simulink model "WF_offshore"  (R2024a)
settings: Solver=VariableStepAuto  StartTime=0  StopTime=1  RelTol=1e-3
values from neighbouring files (symbols this model uses):
  c_c = 0.177e-6    (= 1.77e-07)    [WF_onshore_SSO_GFL.m]    (also in WF_physical_param_offshore_supersynchronous.m = cable_220(i,6)*1e-9; WF_physical_param_onshore_SSO_020625.m = cable_220(i,6)*1e-9; initialize_params_agg.m)
  c_c_eff = c_c*n_cables    [WF_onshore_SSO_GFL.m]    (also in WF_physical_param_offshore_supersynchronous.m; WF_physical_param_onshore_SSO_020625.m; initialize_params_agg.m)
  cvtr = initialize_NR_VSC_GF(cvtr)    [NR_steadystate_VSC_GF.m]    (also in WF_onshore_SSO_GFL.m = setfield(cvtr,'parameters', p_vary.name,p_vary.val(i)); WF_physical_param_offshore_supersynchronous.m = setfield(cvtr,'parameters', p_vary.name,p_vary.val(i)); WF_physical_param_onshore_SSO_020625.m = setfield(cvtr,'parameters', p_vary.name,p_vary.val(i)); impedance_WT_blackbox.m = base_values(cvtr))
  D_C = 10:4:100    [WF_onshore_SSO_GFL.m]    (also in WF_parameter_variation.m = 10:4:150; WF_physical_param.m = 10:4:150; WF_physical_param_offshore_supersynchronous.m = 50; WF_physical_param_onshore_SSO_020625.m = 50)
  enable_pll = 1    [impedance_WT_agg.m]    (also in initialize_WT_agg.m; initialize_WT_default_gfl.m; initialize_WT_default_offshore_super.m)
  f1 = 50    [WF_onshore_SSO_GFL.m]    (also in WF_physical_param_offshore_supersynchronous.m; WF_physical_param_onshore_SSO_020625.m; initialize_params_agg.m)
  i = 1    [WF_physical_param_offshore_supersynchronous.m]    (also in WF_physical_param_onshore_SSO_020625.m)
  L = inv(R)    [participation_factors_VSC_GF.m]
  l_c = 0.386e-3    (= 0.000386)    [WF_onshore_SSO_GFL.m]    (also in WF_physical_param_offshore_supersynchronous.m = cable_220(i,5)*1e-3; WF_physical_param_onshore_SSO_020625.m = cable_220(i,5)*1e-3; initialize_params_agg.m)
  l_c_eff = l_c/n_cables    [WF_onshore_SSO_GFL.m]    (also in WF_physical_param_offshore_supersynchronous.m; WF_physical_param_onshore_SSO_020625.m; initialize_params_agg.m)
  L_comp = sqrt(2)*l_comp*(Z_b_G/(2*pi*f1))    [WF_physical_param.m]    (also in WF_physical_param_offshore_supersynchronous.m = sqrt(2)*((1/(c_c_eff/2*D_C*2*pi*f1))-(l_tf_wf*(Z_b_G)+(l_c_e; WF_physical_param_onshore_SSO_020625.m = sqrt(2)*((1/(c_c_eff/2*D_C*2*pi*f1))-(l_tf_wf*(Z_b_G)+(l_c_e; initialize_params_agg.m)
  l_OH = 0.2    [WF_onshore_SSO_GFL.m]    (also in WF_physical_param_offshore_supersynchronous.m = 0.1; WF_physical_param_onshore_SSO_020625.m = 0.1; initialize_params_agg.m = 0.1)
  l_tf_wf = tf_params(2,2)    [IM_WF_agg.m]    (also in WF_onshore_SSO_GFL.m = 0.05; WF_physical_param_offshore_supersynchronous.m = 0.05; WF_physical_param_onshore_SSO_020625.m = 0.05; initialize_params_agg.m = 0.05)
  l_tf_wt = tf_params(1,2)    [IM_WF_agg.m]    (also in WF_onshore_SSO_GFL.m = 0.0392; WF_physical_param_offshore_supersynchronous.m = 0.0392; WF_physical_param_onshore_SSO_020625.m = 0.0392; initialize_params_agg.m = 0.0392)
  Lg = p_vary(i)*((Z_b_G/(2*pi*f1)))    [WF_onshore_SSO_GFL.m]    (also in WF_physical_param_offshore_supersynchronous.m; WF_physical_param_onshore_SSO_020625.m; initialize_params_agg.m = 0.1*((Z_b_G/(2*pi*f1))))
  Lg1 = Lg    [WF_physical_param_offshore_supersynchronous.m]    (also in WF_physical_param_onshore_SSO_020625.m)
  Lg2 = Lg    [WF_physical_param_offshore_supersynchronous.m]    (also in WF_physical_param_onshore_SSO_020625.m)
  r_c = 27e-3    (= 0.027)    [WF_onshore_SSO_GFL.m]    (also in WF_physical_param_offshore_supersynchronous.m = cable_220(i,4)*1e-3; WF_physical_param_onshore_SSO_020625.m = cable_220(i,4)*1e-3; initialize_params_agg.m)
  r_c_eff = r_c/n_cables    [WF_onshore_SSO_GFL.m]    (also in WF_physical_param_offshore_supersynchronous.m; WF_physical_param_onshore_SSO_020625.m; initialize_params_agg.m)
  r_diss = .1    (= 0.1)    [WF_physical_param_offshore_supersynchronous.m]    (also in WF_physical_param_onshore_SSO_020625.m; calculate_WF.m; initialize_params_agg.m)
  r_OH = 0.02    [WF_onshore_SSO_GFL.m]    (also in WF_physical_param_offshore_supersynchronous.m = 0.01; WF_physical_param_onshore_SSO_020625.m = 0.01; initialize_params_agg.m)
  r_tf_wf = tf_params(2,1)    [IM_WF_agg.m]    (also in WF_onshore_SSO_GFL.m = 0.005; WF_physical_param_offshore_supersynchronous.m = 0.005; WF_physical_param_onshore_SSO_020625.m = 0.005; initialize_params_agg.m = 0.005)
  r_tf_wt = tf_params(1,1)    [IM_WF_agg.m]    (also in WF_onshore_SSO_GFL.m = 0.0056; WF_physical_param_offshore_supersynchronous.m = 0.0056; WF_physical_param_onshore_SSO_020625.m = 0.0056; initialize_params_agg.m = 0.0056)
  Rg = rg*Z_b_G    [WF_onshore_SSO_GFL.m]    (also in WF_physical_param_offshore_supersynchronous.m; WF_physical_param_onshore_SSO_020625.m; initialize_params_agg.m = 0.01*Z_b_G)
  Sb_WF = (3*1)*5e6    (= 15000000)    [WF_onshore_SSO_GFL.m]    (also in WF_physical_param_offshore_supersynchronous.m; WF_physical_param_onshore_SSO_020625.m; impedance_WT_blackbox.m = n_t*Sb_WT; initialize_params_agg.m = 1000000000)
  Sb_WT = 5e6    (= 5000000)    [IM_WF.m]    (also in WF_onshore_SSO_GFL.m; WF_physical_param_offshore_supersynchronous.m; WF_physical_param_onshore_SSO_020625.m; initialize_params_agg.m)
  selector_current_reference = 3    [impedance_WT_agg.m]    (also in initialize_WT_agg.m; initialize_WT_default_gfl.m; initialize_WT_default_offshore_super.m)
  selector_omega_reference = 1    [impedance_WT_agg.m]    (also in initialize_WT_agg.m; initialize_WT_default_gfl.m; initialize_WT_default_offshore_super.m)
  V_coll = 33e3    (= 33000)    [WF_onshore_SSO_GFL.m]    (also in WF_physical_param_offshore_supersynchronous.m; WF_physical_param_onshore_SSO_020625.m; initialize_params_agg.m)
  V_trans = 220e3    (= 220000)    [WF_onshore_SSO_GFL.m]    (also in WF_physical_param_offshore_supersynchronous.m; WF_physical_param_onshore_SSO_020625.m; initialize_params_agg.m)
  Z_b_G = (V_trans/sqrt(3/2))^2/Sb_WF    [WF_onshore_SSO_GFL.m]    (also in WF_physical_param_offshore_supersynchronous.m = (V_b_trans)^2/Sb_WF; WF_physical_param_onshore_SSO_020625.m = (V_b_trans)^2/Sb_WF; initialize_params_agg.m = (V_b_trans)^2/Sb_WF)
undefined symbols (not defined in the file or in its folder): opts, R
libraries: spsSeriesRLCBranchLib x105, simulink_extras x104, simulink x52, spsThreePhaseVIMeasurementLib x42, spsControlledVoltageSourceLib x42, spsGroundLib x41, spsThreePhaseTransformerTwoWindingsLib x14, powerlib_extras x13, spsVariableInductorLib x9, spsIdealSwitchLib x6, spsVariableCapacitorLib x6, spsThreePhaseSeriesRLCBranchLib x4
(part 1 of 13)
settings Model: Creator=andrsmit  LastModifiedBy=andrsmit
settings DataIOCC: InitialState=op.xFinal  SaveFinalState=on  SaveOperatingPoint=on

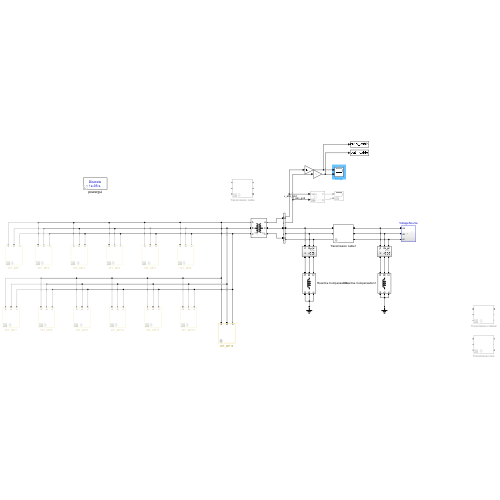
[thumbnail: Simulink's stored preview of the top-level diagram]
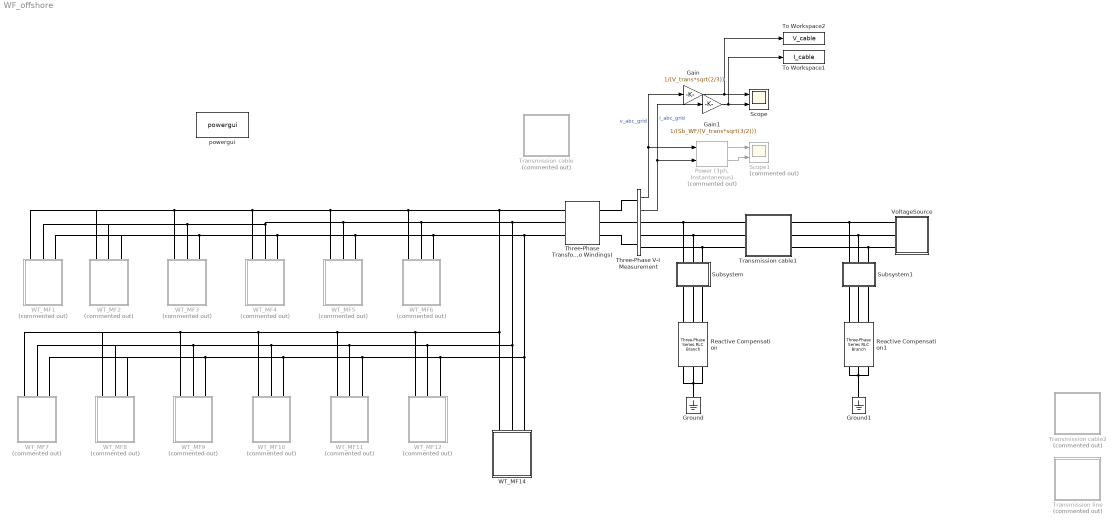
== system WF_offshore ==
  Gain : Gain  Gain=1/(V_trans*sqrt(2/3))
  Gain1 : Gain  Gain=1/(Sb_WF/(V_trans*sqrt(3/2)))
  Ground : spsGroundLib/Ground  LConnTagsString=a
  Ground1 : spsGroundLib/Ground  LConnTagsString=a
  "Power (3ph, Instantaneous)" : spsPower3phInstantaneousLib/Power (3ph, Instantaneous)  Commented=on
  Reactive Compensation : spsThreePhaseSeriesRLCBranchLib/Three-Phase Series RLC Branch  LConnTagsString=A|B|C  RConnTagsString=A|B|C  BranchType=L  Resistance=100  Inductance=L_comp  Capacitance=1e-6  Measurements=None
  Reactive Compensation1 : spsThreePhaseSeriesRLCBranchLib/Three-Phase Series RLC Branch  LConnTagsString=A|B|C  RConnTagsString=A|B|C  BranchType=L  Resistance=100  Inductance=L_comp  Capacitance=1e-6  Measurements=None
  Scope : Scope  NumInputPorts=2
  Scope1 : Scope  Commented=on  NumInputPorts=2
  Subsystem : Subsystem
  Subsystem1 : Subsystem
  Three-Phase Transformer (Two Windings) : spsThreePhaseTransformerTwoWindingsLib/Three-Phase Transformer (Two Windings)  Winding1Connection=Yg  Winding2Connection=Yg  CoreType=Three single-phase transformers  SetSaturation=off  Hysteresis=off  DataFile='hysteresis'  SetInitialFlux=off  Measurements=None  UNITS=pu  NominalPower=[Sb_WF , 50 ]  Winding1=[V_coll , r_tf_wf/2, l_tf_wf/2]  Winding2=[V_trans, r_tf_wf/2, l_tf_wf/2]  Rm=5000  Lm=0  L0=0.5  Saturation=[ 0,0 ; 0.0024,1.2 ; 1.0,1.52 ]  InitialFluxes=[ 0.8 , -0.8 , 0.7 ]  BreakLoop=off  DiscreteSolver=Trapezoidal iterative  DataType=off  TransfoNumber=1
  Three-Phase V-I Measurement : spsThreePhaseVIMeasurementLib/Three-Phase V-I Measurement  VoltageMeasurement=phase-to-ground  SetLabelV=off  LabelV=Vabc  Vpu=off  VpuLL=off  CurrentMeasurement=yes  SetLabelI=off  LabelI=Iabc  Ipu=off  Pbase=100e6  Vbase=500e3  OutputType=Complex  PhasorSimulation=off  PSBequivalent=0
  To Workspace1 : ToWorkspace  VariableName=I_cable  SaveFormat=Structure With Time  SampleTime=-1
      settings: MaxDataPoints=1e5
  To Workspace2 : ToWorkspace  VariableName=V_cable  SaveFormat=Structure With Time  SampleTime=-1
      settings: MaxDataPoints=1e6
  Transmission cable : Subsystem  Commented=on  mask{D=D_C, r=r_c, l=l_c, c=c_c}
      mask prompts: D "Distance (km)"; r "Resistance/km (Ohms/km)"; l "Inductance/km (H/km)"; c "Capacitance/km (F/km)"
      mask DialogControl DescTextVar Prompt: Single PI-line cable model, with no coupling/connection between phases
  Transmission cable1 : Subsystem  mask{D=D_C, r=r_c_eff, l=l_c_eff, c=c_c_eff}
      mask prompts: D "Distance (km)"; r "Resistance/km (Ohms/km)"; l "Inductance/km (H/km)"; c "Capacitance/km (F/km)"
      mask DialogControl DescTextVar Prompt: Single PI-line cable model, with no coupling/connection between phases
  Transmission cable2 : Subsystem  Commented=on  mask{D=D_C, r=r_c_eff, l=l_c_eff, c=c_c_eff}
      mask prompts: D "Distance (km)"; r "Resistance/km (Ohms/km)"; l "Inductance/km (H/km)"; c "Capacitance/km (F/km)"
      mask DialogControl DescTextVar Prompt: Single PI-line cable model, with no coupling/connection between phases
  Transmission line : Subsystem  Commented=on  mask{r=r_OH*Z_b_G, l=l_OH*(Z_b_G/(2*pi*f1))}
      mask prompts: r "Resistance (Ohms)"; l "Inductance (H)"
      mask DialogControl DescTextVar Prompt: Single PI-line cable model, with no coupling/connection between phases
  VoltageSource : Subsystem
  WT_MF1 : Subsystem  Commented=on  mask{cvtr=cvtr}
      mask prompts: cvtr "converter name"
  WT_MF10 : Subsystem  Commented=on  mask{cvtr=cvtr}
      mask prompts: cvtr "converter name"
  WT_MF11 : Subsystem  Commented=on  mask{cvtr=cvtr}
      mask prompts: cvtr "converter name"
  WT_MF12 : Subsystem  Commented=on  mask{cvtr=cvtr}
      mask prompts: cvtr "converter name"
  WT_MF14 : Subsystem  mask{cvtr=cvtr}
      mask prompts: cvtr "converter name"
  WT_MF2 : Subsystem  Commented=on  mask{cvtr=cvtr}
      mask prompts: cvtr "converter name"
  WT_MF3 : Subsystem  Commented=on  mask{cvtr=cvtr}
      mask prompts: cvtr "converter name"
  WT_MF4 : Subsystem  Commented=on  mask{cvtr=cvtr}
      mask prompts: cvtr "converter name"
  WT_MF5 : Subsystem  Commented=on  mask{cvtr=cvtr}
      mask prompts: cvtr "converter name"
  WT_MF6 : Subsystem  Commented=on  mask{cvtr=cvtr}
      mask prompts: cvtr "converter name"
  WT_MF7 : Subsystem  Commented=on  mask{cvtr=cvtr}
      mask prompts: cvtr "converter name"
  WT_MF8 : Subsystem  Commented=on  mask{cvtr=cvtr}
      mask prompts: cvtr "converter name"
  WT_MF9 : Subsystem  Commented=on  mask{cvtr=cvtr}
      mask prompts: cvtr "converter name"
  powergui : spspowerguiLib/powergui  Priority=2  SimulationMode=Discrete  SampleTime=cvtr.parameters.Ts  frequency=60  Iterations=50  frequencyindice=0  Pbase=100e6  ErrMax=0.0001  UnitsV=kV  UnitsW=MW  buscounter=0  FunctionMessages=off  echomessages=off  EnableUseOfTLC=off  CurrentSourceSwitches=off  DisableSnubberDevices=off  DisableRonSwitches=off  DisableVfSwitches=off  DisplayEquations=off  AutomaticDiscreteSolvers=off  SolverType=Tustin  Interpol=off  ExternalGateDelay=off  methode=off  Ts=0  x0status=blocks  SPID=off  SwTol=0  HookPort=off  NonlinearTolerance=1e-4  nMaxIteration=100  ContinueOnMaxIteration=off  RestoreLinks=warning  ResistiveCurrentMeasurement=off  Frange=logspace(0,3,50)  Ylog=off  Xlog=off  ShowGrid=off  save=off  variable=ZData  structure=0  ZoomFFT=on  StartTime=0.0  cycles=1  DisplayStyle=1  fundamental=60  FreqAxis=off  MaxFrequency=1000  frequencyindicesteady=1  RmsSteady=1  display=off
  wires:
  Three-Phase V-I Measurement/1 -> Gain/1, "Power (3ph, Instantaneous)"/1  "v_abc_grid"
  Three-Phase V-I Measurement/2 -> "Power (3ph, Instantaneous)"/2, Gain1/1  "i_abc_grid"
  Gain/1 -> To Workspace2/1, Scope/1
  Gain1/1 -> To Workspace1/1, Scope/2
  "Power (3ph, Instantaneous)"/1 -> Scope1/1
  "Power (3ph, Instantaneous)"/2 -> Scope1/2
  connections:
  Three-Phase Transformer (Two Windings)/RConn1 -- Three-Phase V-I Measurement/LConn1
  Three-Phase Transformer (Two Windings)/RConn2 -- Three-Phase V-I Measurement/LConn2
  Three-Phase Transformer (Two Windings)/RConn3 -- Three-Phase V-I Measurement/LConn3
  WT_MF4/RConn1 -- WT_MF3/RConn1 -- WT_MF2/RConn1 -- WT_MF1/RConn1 -- WT_MF5/RConn1 -- WT_MF6/RConn1 -- WT_MF12/RConn1 -- WT_MF11/RConn1 -- WT_MF10/RConn1 -- WT_MF9/RConn1 -- WT_MF7/RConn1 -- WT_MF8/RConn1 -- WT_MF14/RConn1 -- Three-Phase Transformer (Two Windings)/LConn1
  WT_MF4/RConn2 -- WT_MF3/RConn2 -- WT_MF2/RConn2 -- WT_MF1/RConn2 -- WT_MF5/RConn2 -- WT_MF6/RConn2 -- Three-Phase Transformer (Two Windings)/LConn2 -- WT_MF14/RConn2 -- WT_MF12/RConn2 -- WT_MF11/RConn2 -- WT_MF10/RConn2 -- WT_MF9/RConn2 -- WT_MF7/RConn2 -- WT_MF8/RConn2
  Three-Phase Transformer (Two Windings)/LConn3 -- WT_MF14/RConn3 -- WT_MF12/RConn3 -- WT_MF11/RConn3 -- WT_MF10/RConn3 -- WT_MF9/RConn3 -- WT_MF7/RConn3 -- WT_MF8/RConn3 -- WT_MF6/RConn3 -- WT_MF5/RConn3 -- WT_MF4/RConn3 -- WT_MF3/RConn3 -- WT_MF2/RConn3 -- WT_MF1/RConn3
  Transmission cable1/RConn1 -- Subsystem1/LConn1 -- VoltageSource/RConn1
  VoltageSource/RConn2 -- Subsystem1/LConn2 -- Transmission cable1/RConn2
  Transmission cable1/LConn3 -- Subsystem/LConn3 -- Three-Phase V-I Measurement/RConn3
  Ground/LConn1 -- Reactive Compensation/RConn1 -- Reactive Compensation/RConn3 -- Reactive Compensation/RConn2
  Reactive Compensation1/RConn3 -- Reactive Compensation1/RConn1 -- Ground1/LConn1 -- Reactive Compensation1/RConn2
  Transmission cable1/RConn3 -- Subsystem1/LConn3 -- VoltageSource/RConn3
  Subsystem/RConn2 -- Reactive Compensation/LConn2
  Subsystem/RConn1 -- Reactive Compensation/LConn1
  Transmission cable1/LConn2 -- Subsystem/LConn2 -- Three-Phase V-I Measurement/RConn2
  Subsystem/RConn3 -- Reactive Compensation/LConn3
  Transmission cable1/LConn1 -- Three-Phase V-I Measurement/RConn1 -- Subsystem/LConn1
  Subsystem1/RConn3 -- Reactive Compensation1/LConn3
  Subsystem1/RConn1 -- Reactive Compensation1/LConn1
  Subsystem1/RConn2 -- Reactive Compensation1/LConn2

== system WF_offshore/Subsystem ==
  Ideal Switch : spsIdealSwitchLib/Ideal Switch  Ron=R_comp  Lon=0  IC=0  Rs=r_diss*Z_b_G  Cs=inf  Measurements=off
  Ideal Switch1 : spsIdealSwitchLib/Ideal Switch  Ron=R_comp  Lon=0  IC=0  Rs=r_diss*Z_b_G  Cs=inf  Measurements=off
  Ideal Switch2 : spsIdealSwitchLib/Ideal Switch  Ron=R_comp  Lon=0  IC=0  Rs=r_diss*Z_b_G  Cs=inf  Measurements=off
  Step : Step  Time=0.5  SampleTime=0
  Three-Phase Series RLC Branch : spsThreePhaseSeriesRLCBranchLib/Three-Phase Series RLC Branch  Commented=on  LConnTagsString=A|B|C  RConnTagsString=A|B|C  BranchType=RLC  Resistance=1  Inductance=1e-3  Capacitance=1e-6  Measurements=None
  " A" : PMIOPort  Side=Left
  " B" : PMIOPort  Port=2  Side=Left
  " C" : PMIOPort  Port=3  Side=Left
  "  a" : PMIOPort  Port=4  Side=Right
  "  b" : PMIOPort  Port=5  Side=Right
  "  c" : PMIOPort  Port=6  Side=Right
  wires:
  Step/1 -> Ideal Switch2/1, Ideal Switch1/1, Ideal Switch/1
  connections:
  "  a"/RConn1 -- Ideal Switch/RConn1
  Ideal Switch2/LConn1 -- " C"/RConn1
  Ideal Switch2/RConn1 -- "  c"/RConn1
  " A"/RConn1 -- Ideal Switch/LConn1
  Ideal Switch1/RConn1 -- "  b"/RConn1
  Ideal Switch1/LConn1 -- " B"/RConn1

== system WF_offshore/Subsystem1 ==
  Ideal Switch : spsIdealSwitchLib/Ideal Switch  Ron=R_comp  Lon=0  IC=0  Rs=r_diss*Z_b_G  Cs=inf  Measurements=off
  Ideal Switch1 : spsIdealSwitchLib/Ideal Switch  Ron=R_comp  Lon=0  IC=0  Rs=r_diss*Z_b_G  Cs=inf  Measurements=off
  Ideal Switch2 : spsIdealSwitchLib/Ideal Switch  Ron=R_comp  Lon=0  IC=0  Rs=r_diss*Z_b_G  Cs=inf  Measurements=off
  Step : Step  Time=0.5  Before=1  SampleTime=0
  Three-Phase Series RLC Branch : spsThreePhaseSeriesRLCBranchLib/Three-Phase Series RLC Branch  Commented=on  LConnTagsString=A|B|C  RConnTagsString=A|B|C  BranchType=RLC  Resistance=1  Inductance=1e-3  Capacitance=1e-6  Measurements=None
  " A" : PMIOPort  Side=Left
  " B" : PMIOPort  Port=2  Side=Left
  " C" : PMIOPort  Port=3  Side=Left
  "  a" : PMIOPort  Port=4  Side=Right
  "  b" : PMIOPort  Port=5  Side=Right
  "  c" : PMIOPort  Port=6  Side=Right
  wires:
  Step/1 -> Ideal Switch/1, Ideal Switch1/1, Ideal Switch2/1
  connections:
  Ideal Switch1/LConn1 -- " B"/RConn1
  Ideal Switch1/RConn1 -- "  b"/RConn1
  " A"/RConn1 -- Ideal Switch/LConn1
  Ideal Switch2/RConn1 -- "  c"/RConn1
  Ideal Switch2/LConn1 -- " C"/RConn1
  "  a"/RConn1 -- Ideal Switch/RConn1

== system WF_offshore/Transmission cable ==
  Pi Section Line : spsPiSectionLineLib/Pi Section Line  LConnTagsString=1  RConnTagsString=1  Phases=1  PiSections=1  Length=D  Frequency=50  Resistance=r  Inductance=l  Capacitance=c  SpecifyConductance=off  Conductance=0  Measurements=None  Measurements2=None
      settings: LibrarySourceBlock=sps_lib/Power Grid Elements/Pi Section Line
  Pi Section Line1 : spsPiSectionLineLib/Pi Section Line  LConnTagsString=1  RConnTagsString=1  Phases=1  PiSections=1  Length=D  Frequency=50  Resistance=r  Inductance=l  Capacitance=c  SpecifyConductance=off  Conductance=0  Measurements=None  Measurements2=None
      settings: LibrarySourceBlock=sps_lib/Power Grid Elements/Pi Section Line
  Pi Section Line2 : spsPiSectionLineLib/Pi Section Line  LConnTagsString=1  RConnTagsString=1  Phases=1  PiSections=1  Length=D  Frequency=50  Resistance=r  Inductance=l  Capacitance=c  SpecifyConductance=off  Conductance=0  Measurements=None  Measurements2=None
      settings: LibrarySourceBlock=sps_lib/Power Grid Elements/Pi Section Line
  A : PMIOPort  Side=Left
  a : PMIOPort  Port=2  Side=Right
  B : PMIOPort  Port=3  Side=Left
  b : PMIOPort  Port=4  Side=Right
  C : PMIOPort  Port=5  Side=Left
  c : PMIOPort  Port=6  Side=Right
  connections:
  Pi Section Line2/LConn1 -- C/RConn1
  Pi Section Line1/RConn1 -- b/RConn1
  Pi Section Line2/RConn1 -- c/RConn1
  Pi Section Line1/LConn1 -- B/RConn1
  Pi Section Line/LConn1 -- A/RConn1
  a/RConn1 -- Pi Section Line/RConn1

== system WF_offshore/Transmission cable1 ==
  Subsystem : Subsystem
  Subsystem1 : Subsystem
  Subsystem2 : Subsystem
  A : PMIOPort  Side=Left
  a : PMIOPort  Port=2  Side=Right
  B : PMIOPort  Port=3  Side=Left
  b : PMIOPort  Port=4  Side=Right
  C : PMIOPort  Port=5  Side=Left
  c : PMIOPort  Port=6  Side=Right
  connections:
  Subsystem/RConn1 -- a/RConn1
  Subsystem/LConn1 -- A/RConn1
  Subsystem1/LConn1 -- B/RConn1
  Subsystem2/RConn1 -- c/RConn1
  Subsystem1/RConn1 -- b/RConn1
  Subsystem2/LConn1 -- C/RConn1

== system WF_offshore/Transmission cable2 ==
  Subsystem : Subsystem
  Subsystem1 : Subsystem
  Subsystem2 : Subsystem
  A : PMIOPort  Side=Left
  a : PMIOPort  Port=2  Side=Right
  B : PMIOPort  Port=3  Side=Left
  b : PMIOPort  Port=4  Side=Right
  C : PMIOPort  Port=5  Side=Left
  c : PMIOPort  Port=6  Side=Right
  connections:
  Subsystem2/LConn1 -- C/RConn1
  Subsystem1/RConn1 -- b/RConn1
  Subsystem2/RConn1 -- c/RConn1
  Subsystem1/LConn1 -- B/RConn1
  Subsystem/LConn1 -- A/RConn1
  Subsystem/RConn1 -- a/RConn1

== system WF_offshore/Transmission line ==
  Series RLC Branch1 : spsSeriesRLCBranchLib/Series RLC Branch  LConnTagsString=__new0  RConnTagsString=__new0  BranchType=RL  Resistance=r  Inductance=l  SetiL0=off  InitialCurrent=0  Capacitance=1e-6  Setx0=off  InitialVoltage=0  Measurements=None
  Series RLC Branch3 : spsSeriesRLCBranchLib/Series RLC Branch  LConnTagsString=__new0  RConnTagsString=__new0  BranchType=RL  Resistance=r  Inductance=l  SetiL0=off  InitialCurrent=0  Capacitance=1e-6  Setx0=off  InitialVoltage=0  Measurements=None
  Series RLC Branch4 : spsSeriesRLCBranchLib/Series RLC Branch  LConnTagsString=__new0  RConnTagsString=__new0  BranchType=RL  Resistance=r  Inductance=l  SetiL0=off  InitialCurrent=0  Capacitance=1e-6  Setx0=off  InitialVoltage=0  Measurements=None
  A : PMIOPort  Side=Left
  a : PMIOPort  Port=2  Side=Right
  B : PMIOPort  Port=3  Side=Left
  b : PMIOPort  Port=4  Side=Right
  C : PMIOPort  Port=5  Side=Left
  c : PMIOPort  Port=6  Side=Right
  connections:
  Series RLC Branch1/LConn1 -- a/RConn1
  B/RConn1 -- Series RLC Branch3/RConn1
  Series RLC Branch4/LConn1 -- c/RConn1
  Series RLC Branch3/LConn1 -- b/RConn1
  C/RConn1 -- Series RLC Branch4/RConn1
  A/RConn1 -- Series RLC Branch1/RConn1

== system WF_offshore/VoltageSource ==
  1 : spsThreePhaseVIMeasurementLib/Three-Phase V-I Measurement  VoltageMeasurement=phase-to-ground  SetLabelV=off  LabelV=Vabc_1  Vpu=off  VpuLL=off  CurrentMeasurement=yes  SetLabelI=off  LabelI=Iabc_1  Ipu=off  Pbase=100e6  Vbase=Bus(1,2)*1e3  OutputType=Complex  PhasorSimulation=off  PSBequivalent=0
  40 : spsThreePhaseVIMeasurementLib/Three-Phase V-I Measurement  VoltageMeasurement=phase-to-ground  SetLabelV=off  LabelV=Vabc_1  Vpu=off  VpuLL=off  CurrentMeasurement=yes  SetLabelI=off  LabelI=Iabc_1  Ipu=off  Pbase=100e6  Vbase=Bus(1,2)*1e3  OutputType=Complex  PhasorSimulation=off  PSBequivalent=0
  Add2 : Sum
  Add4 : Sum
  Add5 : Sum
  Gain : Gain  Commented=on  Gain=1/(V_trans*sqrt(2/3))
  Gain1 : Gain  Gain=cvtr.pu.Omegab
  Gain2 : Gain  Commented=on  Gain=1/(Sb_WF/(V_trans*sqrt(3/2)))
  Gain3 : Gain  Commented=on  Gain=1/(V_trans*sqrt(2/3))
  Gain4 : Gain  Commented=on  Gain=1/(Sb_WF/(V_trans*sqrt(3/2)))
  Integrator2 : Integrator  InitialConditionSource=external
  Inverse Park1 : Subsystem
  "Power (3ph, Instantaneous)" : spsPower3phInstantaneousLib/Power (3ph, Instantaneous)
  "Power (3ph, Instantaneous)1" : spsPower3phInstantaneousLib/Power (3ph, Instantaneous)  Commented=on
  Product2 : Product
  Product3 : Product
  Scope : Scope  Commented=on  NumInputPorts=2
  Scope1 : Scope  NumInputPorts=2
  Scope2 : Scope  Commented=on  NumInputPorts=2
  Scope3 : Scope  Commented=on  NumInputPorts=2
  Sine Wave1 : Sin  Commented=on  Amplitude=0.01  Frequency=20*2*pi  SampleTime=0
  Step1 : Step  Commented=on  Time=0.1  After=1e-4  SampleTime=0
  Subsystem1 : Subsystem
  Subsystem2 : Subsystem
  Sum2 : Sum  Inputs=++|
  Sum3 : Sum  Inputs=|++
  To Workspace5 : ToWorkspace  Commented=on  VariableName=V_g  SaveFormat=Structure With Time  SampleTime=-1
      settings: MaxDataPoints=2000000
  To Workspace6 : ToWorkspace  Commented=on  VariableName=I_g  SaveFormat=Structure With Time  SampleTime=-1
      settings: MaxDataPoints=2000000
  d_input1 : Constant  Value=0  SampleTime=opts.inp.ts
  delta1 : Constant  Value=0
  dvnd1 : Constant  Value=0  SampleTime=opts.inp.ts
  dvnq1 : Constant  Value=0  SampleTime=opts.inp.ts
  grid inductance : Subsystem  Commented=on
  grid inductance+line : Subsystem  Commented=on
  grid inductance1 : Subsystem  Commented=on
  grid inductance2 : Subsystem
  io5 : Constant  Value=cvtr.ss.vnd0
  io6 : Constant  Value=V_trans*sqrt(2/3)
  io7 : Constant  Value=cvtr.ss.vnq0
  io8 : Constant  Value=1i
  io9 : Constant  Commented=on  Value=cvtr.pu.Vb*(cvtr.ss.vnd0+i*cvtr.ss.vnq0)
  w1 : Constant  Value=cvtr.parameters.Omegag*cvtr.pu.Omegab
  va : PMIOPort  Side=Right
  vb : PMIOPort  Port=2  Side=Right
  vc : PMIOPort  Port=3  Side=Right
  tag scope: d_input=global, dvnd=global, dvnq=global
  wires:
  40/2 -> Gain2/1, To Workspace6/1, "Power (3ph, Instantaneous)"/2
  40/1 -> Gain/1, To Workspace5/1, "Power (3ph, Instantaneous)"/1
  Integrator2/1 -> Inverse Park1/2(delta)
  io5/1 -> Add5/2  "vnd0"
  Add4/1 -> Product3/1  "vnq"
  Subsystem2/1(x_dq) -> Inverse Park1/1(x_dq)
  Add2/1 -> Integrator2/1
  Inverse Park1/1(x_abc) -> Subsystem1/1(v_abc)
  Step1/1 -> Sum3/1
  Sum2/1 -> Product2/1
  io7/1 -> Add4/2  "vnq0"
  w1/1 -> Add2/1
  Sum3/1 -> [d_input], Gain1/1
  dvnq1/1 -> [dvnq], Add4/1  "dvnq"
  Add5/1 -> Sum2/1  "vnd"
  delta1/1 -> Integrator2/2
  dvnd1/1 -> Add5/1, [dvnd]  "dvnd"
  d_input1/1 -> Sum3/2  "d_inp"
  Product2/1 -> Subsystem2/1(x_d+ix_q)
  io8/1 -> Product3/2
  io6/1 -> Product2/2
  Product3/1 -> Sum2/2
  Gain1/1 -> Add2/2
  Gain/1 -> Scope/1
  Gain2/1 -> Scope/2
  "Power (3ph, Instantaneous)"/1 -> Scope1/1
  "Power (3ph, Instantaneous)"/2 -> Scope1/2
  "Power (3ph, Instantaneous)1"/1 -> Scope2/1
  "Power (3ph, Instantaneous)1"/2 -> Scope2/2
  1/1 -> Gain3/1, "Power (3ph, Instantaneous)1"/1
  1/2 -> Gain4/1, "Power (3ph, Instantaneous)1"/2
  Gain3/1 -> Scope3/1
  Gain4/1 -> Scope3/2
  connections:
  40/LConn1 -- vc/RConn1
  40/LConn2 -- vb/RConn1
  40/LConn3 -- va/RConn1
  grid inductance2/LConn1 -- 40/RConn3
  grid inductance2/LConn2 -- 40/RConn2
  grid inductance2/LConn3 -- 40/RConn1
  grid inductance2/RConn1 -- 1/LConn3
  grid inductance2/RConn2 -- 1/LConn2
  grid inductance2/RConn3 -- 1/LConn1
  1/RConn3 -- Subsystem1/RConn1
  1/RConn2 -- Subsystem1/RConn2
  1/RConn1 -- Subsystem1/RConn3

== system WF_offshore/WT_MF1 ==
  Control System : Subsystem  mask{Ts_control=cvtr.parameters.T_cont}
      mask prompts: Ts_control "Sample Time"
  Gain1 : Gain  Gain=1/cvtr.pu.Vb
  Gain2 : Gain  Gain=1/cvtr.pu.Ib
  Gain5 : Gain  Gain=cvtr.pu.Vb
  I_conv : ToWorkspace  VariableName=I_conv  SaveFormat=Structure With Time  SampleTime=-1
      settings: MaxDataPoints=1000000
  Inverse Park1 : Subsystem
  Scope2 : Scope  NumInputPorts=2
  Subsystem1 : Subsystem
  Subsystem6 : Subsystem
  Three-Phase Transformer (Two Windings) : spsThreePhaseTransformerTwoWindingsLib/Three-Phase Transformer (Two Windings)  Winding1Connection=Yg  Winding2Connection=Yg  CoreType=Three single-phase transformers  SetSaturation=off  Hysteresis=off  DataFile='hysteresis'  SetInitialFlux=off  Measurements=None  UNITS=pu  NominalPower=[ Sb_WT , f1]  Winding1=[cvtr.parameters.Vnr ,r_tf_wt/2 , l_tf_wt/2]  Winding2=[ V_coll , r_tf_wt/2, l_tf_wt/2]  Rm=5000  Lm=0  L0=0.5  Saturation=[ 0,0 ; 0.0024,1.2 ; 1.0,1.52 ]  InitialFluxes=[ 0.8 , -0.8 , 0.7 ]  BreakLoop=off  DiscreteSolver=Trapezoidal iterative  DataType=off  TransfoNumber=1
  Three-Phase V-I Measurement : spsThreePhaseVIMeasurementLib/Three-Phase V-I Measurement  VoltageMeasurement=phase-to-ground  SetLabelV=off  LabelV=Vabc  Vpu=off  VpuLL=off  CurrentMeasurement=yes  SetLabelI=off  LabelI=Iabc  Ipu=off  Pbase=100e6  Vbase=500e3  OutputType=Complex  PhasorSimulation=off  PSBequivalent=0
  Transformations (pu and dq) : Subsystem
  V_conv : ToWorkspace  VariableName=V_conv  SaveFormat=Structure With Time  SampleTime=-1
      settings: MaxDataPoints=1000000
  filter capacitance1 : Subsystem
      settings: PortSchema="{\"entries\":[{\"content\":{\"sides\":[{\"content\":{\"connectorIds\":[\"LConn1\",\"LConn2\",\"LConn3\"]},\"type\":\"ConnectorPlacement.EquallySpacedRectSide\",\"uuid\":\"e81be3d5-6303-4565-8ca3-afc618f21d70\"},{\"content\":{\"connectorIds\":[],\"side\":\"RIGHT\"},\"type\":\"ConnectorPlacement.EquallySpacedRectSide\",\"uuid\":\"458d9030-e614-487d-87de-3e53be7c7da4\"},{\"content\":{\"connectorIds\":[],\"side\":\"TOP\"},\"type\":\"ConnectorPlacement.EquallySpacedRectSide\",\"uuid\":\"a29d66a0-f095-498d-bb9b-96c7f47699d3\"},{\"content\":{\"connectorIds\":[\"Out1\"],\"side\":\"BOTTOM\"},\"type\":\"ConnectorPlacement.EquallySpacedRectSide\",\"uuid\":\"afc68874-c098-43f5-9b37-53a3b484513b\"}]},\"type\":\"ConnectorPlacement.EquallySpacedConnector\",\"uuid\":\"37f495dd-1c12-4bb8-af72-7ef46bbd951c\"}],\"packageUris\":[\"http://schema.mathworks.com/mf0/Connector/R2020b\"],\"version\":\"1.0\"}"
  filter inductance1 : Subsystem
      settings: PortSchema="{\"entries\":[{\"content\":{\"sides\":[{\"content\":{\"connectorIds\":[\"LConn1\",\"LConn2\",\"LConn3\"]},\"type\":\"ConnectorPlacement.EquallySpacedRectSide\",\"uuid\":\"d3d60048-9578-4fa3-8d11-9c8a66a4b1f9\"},{\"content\":{\"connectorIds\":[\"RConn1\",\"RConn2\",\"RConn3\"],\"side\":\"RIGHT\"},\"type\":\"ConnectorPlacement.EquallySpacedRectSide\",\"uuid\":\"184a2c1d-36ab-46d1-99e4-db01aa31ec94\"},{\"content\":{\"connectorIds\":[\"Out1\"],\"side\":\"TOP\"},\"type\":\"ConnectorPlacement.EquallySpacedRectSide\",\"uuid\":\"db651021-9d7f-4124-8d21-ede853163467\"}]},\"type\":\"ConnectorPlacement.EquallySpacedConnector\",\"uuid\":\"723d0964-19fd-4dbe-91e3-e4ea0bb1cca9\"}],\"packageUris\":[\"http://schema.mathworks.com/mf0/Connector/R2020b\"],\"version\":\"1.0\"}"
  a : PMIOPort  Side=Right
  b : PMIOPort  Port=2  Side=Right
  c : PMIOPort  Port=3  Side=Right
  wires:
  Control System/2(thetavsm) -> [Thetavsm]
  Control System/3(vir) -> [vir]
  Control System/1(thetapll) -> [Thetapll]
  Transformations (pu and dq)/2(il) -> Control System/2(il)  "il"
  Transformations (pu and dq)/1(io) -> Control System/1(io)  "io"
  Transformations (pu and dq)/3(p) -> Control System/3(p)  "p"
  Transformations (pu and dq)/4(q) -> Control System/4(q)  "q"
  Transformations (pu and dq)/5(vo_pll) -> Control System/5(vo_pll)  "vo_pll"
  Transformations (pu and dq)/6(vo) -> Control System/6(vo)  "vo"
  [Thetavsm] -> Transformations (pu and dq)/5(Thetavsm)
  [Thetapll] -> Transformations (pu and dq)/6(Thetapll)
  [vir] -> Gain5/1
  Subsystem6/1(x_dq) -> Inverse Park1/1(x_dq)
  Gain5/1 -> Subsystem6/1(x_d+ix_q)
  Three-Phase V-I Measurement/2 -> Gain2/1, [i_abc_grid]  "i_abc_grid"
  Inverse Park1/1(x_abc) -> Subsystem1/1(v_abc)
  Three-Phase V-I Measurement/1 -> Gain1/1, [v_abc_grid]  "v_abc_grid"
  [Thetavsm] -> Inverse Park1/2(delta)
  filter capacitance1/1(v_abc) -> [v_abc_filt]  "v_abc_filt"
  filter inductance1/1(i_abc) -> [i_abc_filt]  "i_abc_filt"
  [v_abc_grid] -> Transformations (pu and dq)/3(v_abc_grid)
  [v_abc_filt] -> Transformations (pu and dq)/4(v_abc_filt)
  [i_abc_filt] -> Transformations (pu and dq)/2(i_abc_filt)
  [i_abc_grid] -> Transformations (pu and dq)/1(i_abc_grid)
  Gain1/1 -> Scope2/1, V_conv/1
  Gain2/1 -> Scope2/2, I_conv/1
  connections:
  filter inductance1/RConn3 -- filter capacitance1/LConn3 -- Three-Phase V-I Measurement/LConn3
  filter inductance1/RConn1 -- filter capacitance1/LConn1 -- Three-Phase V-I Measurement/LConn1
  filter inductance1/RConn2 -- filter capacitance1/LConn2 -- Three-Phase V-I Measurement/LConn2
  Subsystem1/RConn1 -- filter inductance1/LConn1
  Subsystem1/RConn2 -- filter inductance1/LConn2
  Subsystem1/RConn3 -- filter inductance1/LConn3
  Three-Phase Transformer (Two Windings)/RConn1 -- a/RConn1
  Three-Phase Transformer (Two Windings)/RConn2 -- b/RConn1
  Three-Phase Transformer (Two Windings)/RConn3 -- c/RConn1
  Three-Phase Transformer (Two Windings)/LConn1 -- Three-Phase V-I Measurement/RConn1
  Three-Phase Transformer (Two Windings)/LConn2 -- Three-Phase V-I Measurement/RConn2
  Three-Phase Transformer (Two Windings)/LConn3 -- Three-Phase V-I Measurement/RConn3

== system WF_offshore/WT_MF10 ==
  Control System : Subsystem  mask{Ts_control=cvtr.parameters.T_cont}
      mask prompts: Ts_control "Sample Time"
  Gain5 : Gain  Gain=cvtr.pu.Vb
  Inverse Park1 : Subsystem
  Subsystem1 : Subsystem
  Subsystem6 : Subsystem
  Three-Phase Transformer (Two Windings) : spsThreePhaseTransformerTwoWindingsLib/Three-Phase Transformer (Two Windings)  Winding1Connection=Yg  Winding2Connection=Yg  CoreType=Three single-phase transformers  SetSaturation=off  Hysteresis=off  DataFile='hysteresis'  SetInitialFlux=off  Measurements=None  UNITS=pu  NominalPower=[Sb_WT, f1 ]  Winding1=[ cvtr.parameters.Vnr ,r_tf_wt/2 , l_tf_wt/2]  Winding2=[ V_coll , r_tf_wt/2, l_tf_wt/2]  Rm=5000  Lm=0  L0=0.5  Saturation=[ 0,0 ; 0.0024,1.2 ; 1.0,1.52 ]  InitialFluxes=[ 0.8 , -0.8 , 0.7 ]  BreakLoop=off  DiscreteSolver=Trapezoidal iterative  DataType=off  TransfoNumber=1
  Three-Phase V-I Measurement : spsThreePhaseVIMeasurementLib/Three-Phase V-I Measurement  VoltageMeasurement=phase-to-ground  SetLabelV=off  LabelV=Vabc  Vpu=off  VpuLL=off  CurrentMeasurement=yes  SetLabelI=off  LabelI=Iabc  Ipu=off  Pbase=100e6  Vbase=500e3  OutputType=Complex  PhasorSimulation=off  PSBequivalent=0
  Transformations (pu and dq) : Subsystem
  filter capacitance1 : Subsystem
      settings: PortSchema="{\"entries\":[{\"content\":{\"sides\":[{\"content\":{\"connectorIds\":[\"LConn1\",\"LConn2\",\"LConn3\"]},\"type\":\"ConnectorPlacement.EquallySpacedRectSide\",\"uuid\":\"e81be3d5-6303-4565-8ca3-afc618f21d70\"},{\"content\":{\"connectorIds\":[],\"side\":\"RIGHT\"},\"type\":\"ConnectorPlacement.EquallySpacedRectSide\",\"uuid\":\"458d9030-e614-487d-87de-3e53be7c7da4\"},{\"content\":{\"connectorIds\":[],\"side\":\"TOP\"},\"type\":\"ConnectorPlacement.EquallySpacedRectSide\",\"uuid\":\"a29d66a0-f095-498d-bb9b-96c7f47699d3\"},{\"content\":{\"connectorIds\":[\"Out1\"],\"side\":\"BOTTOM\"},\"type\":\"ConnectorPlacement.EquallySpacedRectSide\",\"uuid\":\"afc68874-c098-43f5-9b37-53a3b484513b\"}]},\"type\":\"ConnectorPlacement.EquallySpacedConnector\",\"uuid\":\"37f495dd-1c12-4bb8-af72-7ef46bbd951c\"}],\"packageUris\":[\"http://schema.mathworks.com/mf0/Connector/R2020b\"],\"version\":\"1.0\"}"
  filter inductance1 : Subsystem
      settings: PortSchema="{\"entries\":[{\"content\":{\"sides\":[{\"content\":{\"connectorIds\":[\"LConn1\",\"LConn2\",\"LConn3\"]},\"type\":\"ConnectorPlacement.EquallySpacedRectSide\",\"uuid\":\"d3d60048-9578-4fa3-8d11-9c8a66a4b1f9\"},{\"content\":{\"connectorIds\":[\"RConn1\",\"RConn2\",\"RConn3\"],\"side\":\"RIGHT\"},\"type\":\"ConnectorPlacement.EquallySpacedRectSide\",\"uuid\":\"184a2c1d-36ab-46d1-99e4-db01aa31ec94\"},{\"content\":{\"connectorIds\":[\"Out1\"],\"side\":\"TOP\"},\"type\":\"ConnectorPlacement.EquallySpacedRectSide\",\"uuid\":\"db651021-9d7f-4124-8d21-ede853163467\"}]},\"type\":\"ConnectorPlacement.EquallySpacedConnector\",\"uuid\":\"723d0964-19fd-4dbe-91e3-e4ea0bb1cca9\"}],\"packageUris\":[\"http://schema.mathworks.com/mf0/Connector/R2020b\"],\"version\":\"1.0\"}"
  a : PMIOPort  Side=Right
  b : PMIOPort  Port=2  Side=Right
  c : PMIOPort  Port=3  Side=Right
  wires:
  [i_abc_grid] -> Transformations (pu and dq)/1(i_abc_grid)
  [i_abc_filt] -> Transformations (pu and dq)/2(i_abc_filt)
  [v_abc_filt] -> Transformations (pu and dq)/4(v_abc_filt)
  [v_abc_grid] -> Transformations (pu and dq)/3(v_abc_grid)
  filter inductance1/1(i_abc) -> [i_abc_filt]  "i_abc_filt"
  filter capacitance1/1(v_abc) -> [v_abc_filt]  "v_abc_filt"
  [Thetavsm] -> Inverse Park1/2(delta)
  Three-Phase V-I Measurement/1 -> [v_abc_grid]  "v_abc_grid"
  Inverse Park1/1(x_abc) -> Subsystem1/1(v_abc)
  Three-Phase V-I Measurement/2 -> [i_abc_grid]  "i_abc_grid"
  Gain5/1 -> Subsystem6/1(x_d+ix_q)
  Subsystem6/1(x_dq) -> Inverse Park1/1(x_dq)
  [vir] -> Gain5/1
  [Thetapll] -> Transformations (pu and dq)/6(Thetapll)
  [Thetavsm] -> Transformations (pu and dq)/5(Thetavsm)
  Transformations (pu and dq)/6(vo) -> Control System/6(vo)  "vo"
  Transformations (pu and dq)/5(vo_pll) -> Control System/5(vo_pll)  "vo_pll"
  Transformations (pu and dq)/4(q) -> Control System/4(q)  "q"
  Transformations (pu and dq)/3(p) -> Control System/3(p)  "p"
  Transformations (pu and dq)/1(io) -> Control System/1(io)  "io"
  Transformations (pu and dq)/2(il) -> Control System/2(il)  "il"
  Control System/1(thetapll) -> [Thetapll]
  Control System/3(vir) -> [vir]
  Control System/2(thetavsm) -> [Thetavsm]
  connections:
  Three-Phase Transformer (Two Windings)/LConn3 -- Three-Phase V-I Measurement/RConn3
  Three-Phase Transformer (Two Windings)/LConn2 -- Three-Phase V-I Measurement/RConn2
  Three-Phase Transformer (Two Windings)/LConn1 -- Three-Phase V-I Measurement/RConn1
  Three-Phase Transformer (Two Windings)/RConn3 -- c/RConn1
  Three-Phase Transformer (Two Windings)/RConn2 -- b/RConn1
  Three-Phase Transformer (Two Windings)/RConn1 -- a/RConn1
  Subsystem1/RConn3 -- filter inductance1/LConn3
  Subsystem1/RConn2 -- filter inductance1/LConn2
  Subsystem1/RConn1 -- filter inductance1/LConn1
  Three-Phase V-I Measurement/LConn2 -- filter capacitance1/LConn2 -- filter inductance1/RConn2
  Three-Phase V-I Measurement/LConn1 -- filter capacitance1/LConn1 -- filter inductance1/RConn1
  Three-Phase V-I Measurement/LConn3 -- filter capacitance1/LConn3 -- filter inductance1/RConn3

== system WF_offshore/WT_MF11 ==
  Control System : Subsystem  mask{Ts_control=cvtr.parameters.T_cont}
      mask prompts: Ts_control "Sample Time"
  Gain5 : Gain  Gain=cvtr.pu.Vb
  Inverse Park1 : Subsystem
  Subsystem1 : Subsystem
  Subsystem6 : Subsystem
  Three-Phase Transformer (Two Windings) : spsThreePhaseTransformerTwoWindingsLib/Three-Phase Transformer (Two Windings)  Winding1Connection=Yg  Winding2Connection=Yg  CoreType=Three single-phase transformers  SetSaturation=off  Hysteresis=off  DataFile='hysteresis'  SetInitialFlux=off  Measurements=None  UNITS=pu  NominalPower=[Sb_WT, f1 ]  Winding1=[ cvtr.parameters.Vnr ,r_tf_wt/2 , l_tf_wt/2]  Winding2=[ V_coll , r_tf_wt/2, l_tf_wt/2]  Rm=5000  Lm=0  L0=0.5  Saturation=[ 0,0 ; 0.0024,1.2 ; 1.0,1.52 ]  InitialFluxes=[ 0.8 , -0.8 , 0.7 ]  BreakLoop=off  DiscreteSolver=Trapezoidal iterative  DataType=off  TransfoNumber=1
  Three-Phase V-I Measurement : spsThreePhaseVIMeasurementLib/Three-Phase V-I Measurement  VoltageMeasurement=phase-to-ground  SetLabelV=off  LabelV=Vabc  Vpu=off  VpuLL=off  CurrentMeasurement=yes  SetLabelI=off  LabelI=Iabc  Ipu=off  Pbase=100e6  Vbase=500e3  OutputType=Complex  PhasorSimulation=off  PSBequivalent=0
  Transformations (pu and dq) : Subsystem
  filter capacitance1 : Subsystem
      settings: PortSchema="{\"entries\":[{\"content\":{\"sides\":[{\"content\":{\"connectorIds\":[\"LConn1\",\"LConn2\",\"LConn3\"]},\"type\":\"ConnectorPlacement.EquallySpacedRectSide\",\"uuid\":\"e81be3d5-6303-4565-8ca3-afc618f21d70\"},{\"content\":{\"connectorIds\":[],\"side\":\"RIGHT\"},\"type\":\"ConnectorPlacement.EquallySpacedRectSide\",\"uuid\":\"458d9030-e614-487d-87de-3e53be7c7da4\"},{\"content\":{\"connectorIds\":[],\"side\":\"TOP\"},\"type\":\"ConnectorPlacement.EquallySpacedRectSide\",\"uuid\":\"a29d66a0-f095-498d-bb9b-96c7f47699d3\"},{\"content\":{\"connectorIds\":[\"Out1\"],\"side\":\"BOTTOM\"},\"type\":\"ConnectorPlacement.EquallySpacedRectSide\",\"uuid\":\"afc68874-c098-43f5-9b37-53a3b484513b\"}]},\"type\":\"ConnectorPlacement.EquallySpacedConnector\",\"uuid\":\"37f495dd-1c12-4bb8-af72-7ef46bbd951c\"}],\"packageUris\":[\"http://schema.mathworks.com/mf0/Connector/R2020b\"],\"version\":\"1.0\"}"
  filter inductance1 : Subsystem
      settings: PortSchema="{\"entries\":[{\"content\":{\"sides\":[{\"content\":{\"connectorIds\":[\"LConn1\",\"LConn2\",\"LConn3\"]},\"type\":\"ConnectorPlacement.EquallySpacedRectSide\",\"uuid\":\"d3d60048-9578-4fa3-8d11-9c8a66a4b1f9\"},{\"content\":{\"connectorIds\":[\"RConn1\",\"RConn2\",\"RConn3\"],\"side\":\"RIGHT\"},\"type\":\"ConnectorPlacement.EquallySpacedRectSide\",\"uuid\":\"184a2c1d-36ab-46d1-99e4-db01aa31ec94\"},{\"content\":{\"connectorIds\":[\"Out1\"],\"side\":\"TOP\"},\"type\":\"ConnectorPlacement.EquallySpacedRectSide\",\"uuid\":\"db651021-9d7f-4124-8d21-ede853163467\"}]},\"type\":\"ConnectorPlacement.EquallySpacedConnector\",\"uuid\":\"723d0964-19fd-4dbe-91e3-e4ea0bb1cca9\"}],\"packageUris\":[\"http://schema.mathworks.com/mf0/Connector/R2020b\"],\"version\":\"1.0\"}"
  a : PMIOPort  Side=Right
  b : PMIOPort  Port=2  Side=Right
  c : PMIOPort  Port=3  Side=Right
  wires:
  Control System/2(thetavsm) -> [Thetavsm]
  Control System/3(vir) -> [vir]
  Control System/1(thetapll) -> [Thetapll]
  Transformations (pu and dq)/2(il) -> Control System/2(il)  "il"
  Transformations (pu and dq)/1(io) -> Control System/1(io)  "io"
  Transformations (pu and dq)/3(p) -> Control System/3(p)  "p"
  Transformations (pu and dq)/4(q) -> Control System/4(q)  "q"
  Transformations (pu and dq)/5(vo_pll) -> Control System/5(vo_pll)  "vo_pll"
  Transformations (pu and dq)/6(vo) -> Control System/6(vo)  "vo"
  [Thetavsm] -> Transformations (pu and dq)/5(Thetavsm)
  [Thetapll] -> Transformations (pu and dq)/6(Thetapll)
  [vir] -> Gain5/1
  Subsystem6/1(x_dq) -> Inverse Park1/1(x_dq)
  Gain5/1 -> Subsystem6/1(x_d+ix_q)
  Three-Phase V-I Measurement/2 -> [i_abc_grid]  "i_abc_grid"
  Inverse Park1/1(x_abc) -> Subsystem1/1(v_abc)
  Three-Phase V-I Measurement/1 -> [v_abc_grid]  "v_abc_grid"
  [Thetavsm] -> Inverse Park1/2(delta)
  filter capacitance1/1(v_abc) -> [v_abc_filt]  "v_abc_filt"
  filter inductance1/1(i_abc) -> [i_abc_filt]  "i_abc_filt"
  [v_abc_grid] -> Transformations (pu and dq)/3(v_abc_grid)
  [v_abc_filt] -> Transformations (pu and dq)/4(v_abc_filt)
  [i_abc_filt] -> Transformations (pu and dq)/2(i_abc_filt)
  [i_abc_grid] -> Transformations (pu and dq)/1(i_abc_grid)
  connections:
  filter inductance1/RConn3 -- filter capacitance1/LConn3 -- Three-Phase V-I Measurement/LConn3
  filter inductance1/RConn1 -- filter capacitance1/LConn1 -- Three-Phase V-I Measurement/LConn1
  filter inductance1/RConn2 -- filter capacitance1/LConn2 -- Three-Phase V-I Measurement/LConn2
  Subsystem1/RConn1 -- filter inductance1/LConn1
  Subsystem1/RConn2 -- filter inductance1/LConn2
  Subsystem1/RConn3 -- filter inductance1/LConn3
  Three-Phase Transformer (Two Windings)/RConn1 -- a/RConn1
  Three-Phase Transformer (Two Windings)/RConn2 -- b/RConn1
  Three-Phase Transformer (Two Windings)/RConn3 -- c/RConn1
  Three-Phase Transformer (Two Windings)/LConn1 -- Three-Phase V-I Measurement/RConn1
  Three-Phase Transformer (Two Windings)/LConn2 -- Three-Phase V-I Measurement/RConn2
  Three-Phase Transformer (Two Windings)/LConn3 -- Three-Phase V-I Measurement/RConn3

== system WF_offshore/WT_MF12 ==
  Control System : Subsystem  mask{Ts_control=cvtr.parameters.T_cont}
      mask prompts: Ts_control "Sample Time"
  Gain5 : Gain  Gain=cvtr.pu.Vb
  Inverse Park1 : Subsystem
  Subsystem1 : Subsystem
  Subsystem6 : Subsystem
  Three-Phase Transformer (Two Windings) : spsThreePhaseTransformerTwoWindingsLib/Three-Phase Transformer (Two Windings)  Winding1Connection=Yg  Winding2Connection=Yg  CoreType=Three single-phase transformers  SetSaturation=off  Hysteresis=off  DataFile='hysteresis'  SetInitialFlux=off  Measurements=None  UNITS=pu  NominalPower=[Sb_WT, f1 ]  Winding1=[ cvtr.parameters.Vnr ,r_tf_wt/2 , l_tf_wt/2]  Winding2=[ V_coll , r_tf_wt/2, l_tf_wt/2]  Rm=5000  Lm=0  L0=0.5  Saturation=[ 0,0 ; 0.0024,1.2 ; 1.0,1.52 ]  InitialFluxes=[ 0.8 , -0.8 , 0.7 ]  BreakLoop=off  DiscreteSolver=Trapezoidal iterative  DataType=off  TransfoNumber=1
  Three-Phase V-I Measurement : spsThreePhaseVIMeasurementLib/Three-Phase V-I Measurement  VoltageMeasurement=phase-to-ground  SetLabelV=off  LabelV=Vabc  Vpu=off  VpuLL=off  CurrentMeasurement=yes  SetLabelI=off  LabelI=Iabc  Ipu=off  Pbase=100e6  Vbase=500e3  OutputType=Complex  PhasorSimulation=off  PSBequivalent=0
  Transformations (pu and dq) : Subsystem
  filter capacitance1 : Subsystem
      settings: PortSchema="{\"entries\":[{\"content\":{\"sides\":[{\"content\":{\"connectorIds\":[\"LConn1\",\"LConn2\",\"LConn3\"]},\"type\":\"ConnectorPlacement.EquallySpacedRectSide\",\"uuid\":\"e81be3d5-6303-4565-8ca3-afc618f21d70\"},{\"content\":{\"connectorIds\":[],\"side\":\"RIGHT\"},\"type\":\"ConnectorPlacement.EquallySpacedRectSide\",\"uuid\":\"458d9030-e614-487d-87de-3e53be7c7da4\"},{\"content\":{\"connectorIds\":[],\"side\":\"TOP\"},\"type\":\"ConnectorPlacement.EquallySpacedRectSide\",\"uuid\":\"a29d66a0-f095-498d-bb9b-96c7f47699d3\"},{\"content\":{\"connectorIds\":[\"Out1\"],\"side\":\"BOTTOM\"},\"type\":\"ConnectorPlacement.EquallySpacedRectSide\",\"uuid\":\"afc68874-c098-43f5-9b37-53a3b484513b\"}]},\"type\":\"ConnectorPlacement.EquallySpacedConnector\",\"uuid\":\"37f495dd-1c12-4bb8-af72-7ef46bbd951c\"}],\"packageUris\":[\"http://schema.mathworks.com/mf0/Connector/R2020b\"],\"version\":\"1.0\"}"
  filter inductance1 : Subsystem
      settings: PortSchema="{\"entries\":[{\"content\":{\"sides\":[{\"content\":{\"connectorIds\":[\"LConn1\",\"LConn2\",\"LConn3\"]},\"type\":\"ConnectorPlacement.EquallySpacedRectSide\",\"uuid\":\"d3d60048-9578-4fa3-8d11-9c8a66a4b1f9\"},{\"content\":{\"connectorIds\":[\"RConn1\",\"RConn2\",\"RConn3\"],\"side\":\"RIGHT\"},\"type\":\"ConnectorPlacement.EquallySpacedRectSide\",\"uuid\":\"184a2c1d-36ab-46d1-99e4-db01aa31ec94\"},{\"content\":{\"connectorIds\":[\"Out1\"],\"side\":\"TOP\"},\"type\":\"ConnectorPlacement.EquallySpacedRectSide\",\"uuid\":\"db651021-9d7f-4124-8d21-ede853163467\"}]},\"type\":\"ConnectorPlacement.EquallySpacedConnector\",\"uuid\":\"723d0964-19fd-4dbe-91e3-e4ea0bb1cca9\"}],\"packageUris\":[\"http://schema.mathworks.com/mf0/Connector/R2020b\"],\"version\":\"1.0\"}"
  a : PMIOPort  Side=Right
  b : PMIOPort  Port=2  Side=Right
  c : PMIOPort  Port=3  Side=Right
  wires:
  [i_abc_grid] -> Transformations (pu and dq)/1(i_abc_grid)
  [i_abc_filt] -> Transformations (pu and dq)/2(i_abc_filt)
  [v_abc_filt] -> Transformations (pu and dq)/4(v_abc_filt)
  [v_abc_grid] -> Transformations (pu and dq)/3(v_abc_grid)
  filter inductance1/1(i_abc) -> [i_abc_filt]  "i_abc_filt"
  filter capacitance1/1(v_abc) -> [v_abc_filt]  "v_abc_filt"
  [Thetavsm] -> Inverse Park1/2(delta)
  Three-Phase V-I Measurement/1 -> [v_abc_grid]  "v_abc_grid"
  Inverse Park1/1(x_abc) -> Subsystem1/1(v_abc)
  Three-Phase V-I Measurement/2 -> [i_abc_grid]  "i_abc_grid"
  Gain5/1 -> Subsystem6/1(x_d+ix_q)
  Subsystem6/1(x_dq) -> Inverse Park1/1(x_dq)
  [vir] -> Gain5/1
  [Thetapll] -> Transformations (pu and dq)/6(Thetapll)
  [Thetavsm] -> Transformations (pu and dq)/5(Thetavsm)
  Transformations (pu and dq)/6(vo) -> Control System/6(vo)  "vo"
  Transformations (pu and dq)/5(vo_pll) -> Control System/5(vo_pll)  "vo_pll"
  Transformations (pu and dq)/4(q) -> Control System/4(q)  "q"
  Transformations (pu and dq)/3(p) -> Control System/3(p)  "p"
  Transformations (pu and dq)/1(io) -> Control System/1(io)  "io"
  Transformations (pu and dq)/2(il) -> Control System/2(il)  "il"
  Control System/1(thetapll) -> [Thetapll]
  Control System/3(vir) -> [vir]
  Control System/2(thetavsm) -> [Thetavsm]
  connections:
  Three-Phase Transformer (Two Windings)/LConn3 -- Three-Phase V-I Measurement/RConn3
  Three-Phase Transformer (Two Windings)/LConn2 -- Three-Phase V-I Measurement/RConn2
  Three-Phase Transformer (Two Windings)/LConn1 -- Three-Phase V-I Measurement/RConn1
  Three-Phase Transformer (Two Windings)/RConn3 -- c/RConn1
  Three-Phase Transformer (Two Windings)/RConn2 -- b/RConn1
  Three-Phase Transformer (Two Windings)/RConn1 -- a/RConn1
  Subsystem1/RConn3 -- filter inductance1/LConn3
  Subsystem1/RConn2 -- filter inductance1/LConn2
  Subsystem1/RConn1 -- filter inductance1/LConn1
  Three-Phase V-I Measurement/LConn2 -- filter capacitance1/LConn2 -- filter inductance1/RConn2
  Three-Phase V-I Measurement/LConn1 -- filter capacitance1/LConn1 -- filter inductance1/RConn1
  Three-Phase V-I Measurement/LConn3 -- filter capacitance1/LConn3 -- filter inductance1/RConn3
